simulink model "openLoopCruiseControl_v1"  (R2024a)
settings: Solver=VariableStepAuto  StartTime=0.0  StopTime=200  RelTol=1e-3
values from neighbouring files (symbols this model uses):
  Af = 2.2    [vehicle_data1.m]
  Cd = 0.3    [vehicle_data1.m]
  Cr = 0.015    [vehicle_data1.m]
  gravity = 9.81    [vehicle_data1.m]
  rho = 1.225    [vehicle_data1.m]
  vehicle_mass = 1500    [vehicle_data1.m]
undefined symbols (not defined in the file or in its folder): magnitude
libraries: simulink x1
settings Model: Creator=Sarthak Sahoo  LastModifiedBy=Sarthak Sahoo

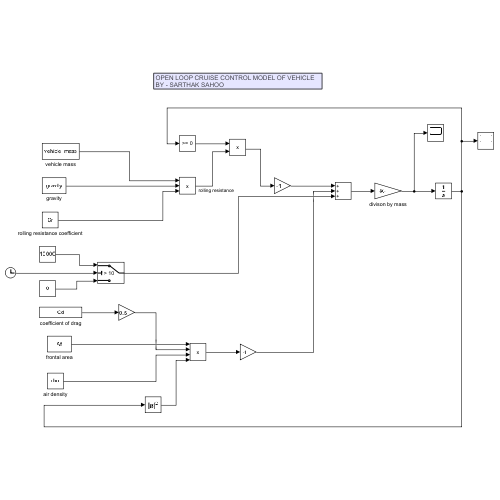
[thumbnail: Simulink's stored preview of the top-level diagram]
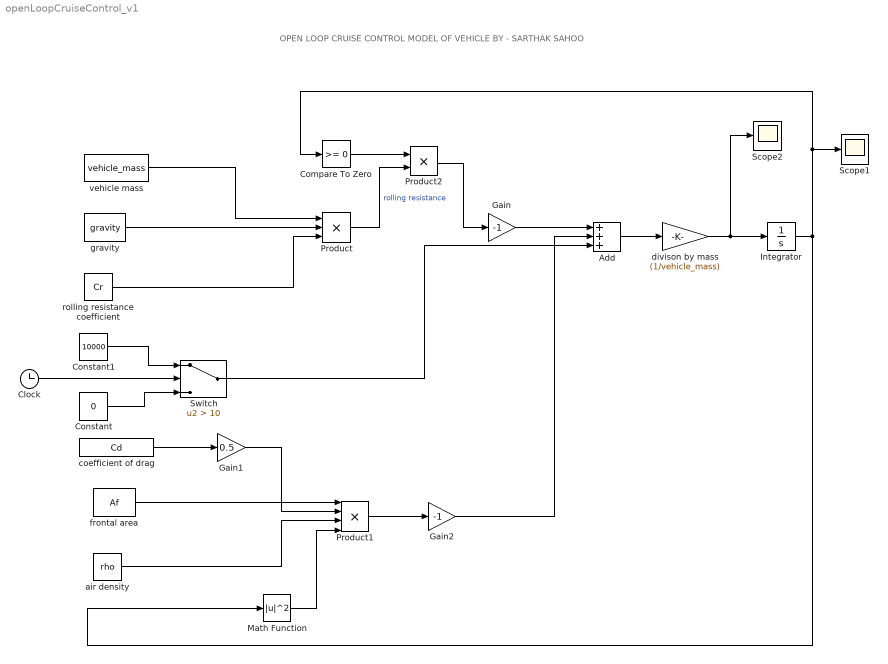
== system openLoopCruiseControl_v1 ==
  note: OPEN LOOP CRUISE CONTROL MODEL OF VEHICLE
      | BY - SARTHAK SAHOO
  Add : Sum  Inputs=+++
  Clock : Clock
  Compare To Zero : simulink/Logic and Bit Operations/Compare To Zero  relop=>=  OutDataTypeStr=boolean
  Constant : Constant  Value=0
  Constant1 : Constant  Value=10000
  Gain : Gain  Gain=-1
  Gain1 : Gain  Gain=0.5
  Gain2 : Gain  Gain=-1
  Integrator : Integrator
  Math Function : Math  Operator=magnitude^2
  Product : Product  Inputs=3
  Product1 : Product  Inputs=4
  Product2 : Product
  Scope1 : Scope
  Scope2 : Scope
  Switch : Switch  Criteria=u2 > Threshold  Threshold=10  SaturateOnIntegerOverflow=off  InputSameDT=off
  air density : Constant  Value=rho
  coefficient of drag : Constant  Value=Cd
  divison by mass : Gain  Gain=(1/vehicle_mass)
  frontal area : Constant  Value=Af
  gravity : Constant  Value=gravity
  rolling resistance coefficient : Constant  Value=Cr
  vehicle mass : Constant  Value=vehicle_mass
  wires:
  vehicle mass/1 -> Product/1
  gravity/1 -> Product/2
  rolling resistance coefficient/1 -> Product/3
  Gain/1 -> Add/1
  air density/1 -> Product1/3
  frontal area/1 -> Product1/1
  coefficient of drag/1 -> Gain1/1
  Gain1/1 -> Product1/2
  Product1/1 -> Gain2/1
  Gain2/1 -> Add/2
  Add/1 -> divison by mass/1
  divison by mass/1 -> Scope2/1, Integrator/1
  Integrator/1 -> Math Function/1, Scope1/1, Compare To Zero/1
  Math Function/1 -> Product1/4
  Constant1/1 -> Switch/1
  Constant/1 -> Switch/3
  Clock/1 -> Switch/2
  Compare To Zero/1 -> Product2/1
  Product/1 -> Product2/2  "rolling resistance"
  Product2/1 -> Gain/1
  Switch/1 -> Add/3
